simulink model "antiwindup_complete_reference"  (R2021a)
settings: Solver=VariableStepAuto  StartTime=0.0  StopTime=1  RelTol=1e-8
settings Model: Creator=cnjones  LastModifiedBy=马骏涛
settings SolverCC: AlgebraicLoopSolver=TrustRegion
settings RTWCC: DLArmComputeVersion=20.02.1

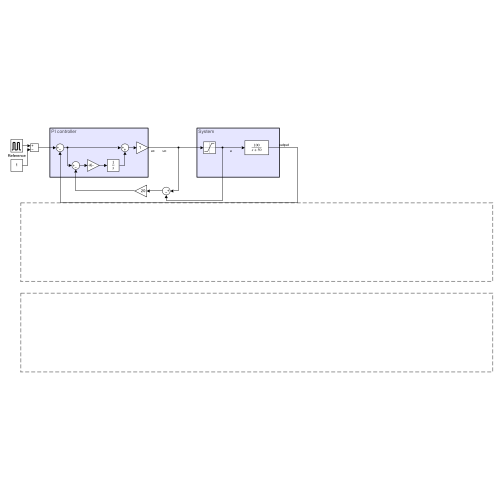
[thumbnail: Simulink's stored preview of the top-level diagram]
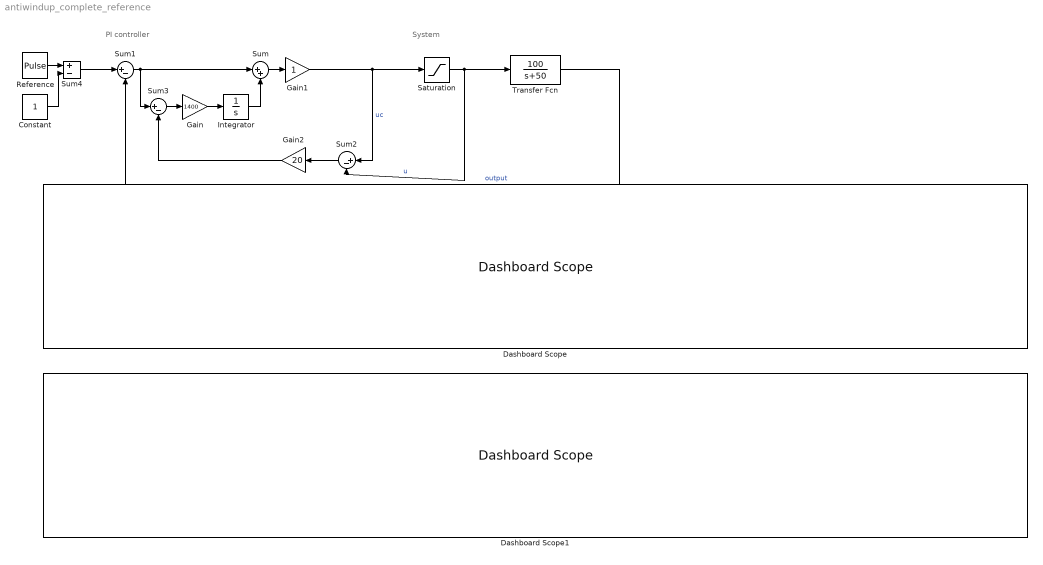
== system antiwindup_complete_reference ==
  note: System
  note: PI controller
  Constant : Constant
  Dashboard Scope : DashboardScope  Ymin=-5  Ymax=5  ScaleAtStop=off
  Dashboard Scope1 : DashboardScope  Ymin=-1  Ymax=2
  Gain : Gain  Gain=1400
  Gain1 : Gain
  Gain2 : Gain  Gain=20
  Integrator : Integrator
  Reference : DiscretePulseGenerator  PulseType=Time based  Amplitude=2  Period=0.25  PulseWidth=50
  Saturation : Saturate  UpperLimit=2  LowerLimit=-2
  Sum : Sum  Inputs=|++
  Sum1 : Sum  Inputs=|+-
  Sum2 : Sum  Inputs=|+-
  Sum3 : Sum  Inputs=|+-
  Sum4 : Sum  Inputs=+-
  Transfer Fcn : TransferFcn  Numerator=100  Denominator=[1 50]
  wires:
  Gain/1 -> Integrator/1
  Sum/1 -> Gain1/1
  Integrator/1 -> Sum/2
  Gain1/1 -> Sum2/1, Saturation/1  "uc"
  Transfer Fcn/1 -> Sum1/2  "output"
  Sum1/1 -> Sum3/1, Sum/1
  Reference/1 -> Sum4/1
  Constant/1 -> Sum4/2
  Sum4/1 -> Sum1/1
  Saturation/1 -> Sum2/2, Transfer Fcn/1  "u"
  Sum2/1 -> Gain2/1
  Sum3/1 -> Gain/1
  Gain2/1 -> Sum3/2
